simulink model "N3Z_tonetestNotWorking"  (R2014b)
settings: Solver=ode3  SolverMode=SingleTasking  StartTime=0.0  StopTime=1e-4  FixedStep=fpgaclk  RelTol=1e-3
PreLoadFcn:
  | %fpgaclk=1/32.768e6
  | fpgaclk=1/49.162e6
  | 
  | SerialData=[1,zeros(1,11),1,0,0,1]
  | load ../N3workingG/window
  | win=win';  %Go back to using flatter and wider windowed sync function
  | %load ../N3workingG/hanning    %use Hahn window
  | 
  | load ../N3workingG/PREemphasis   %For pre-empasis and deemphasis FIRs
  | 
  | %LUT3=xls2LUT2('../IQI_Qdemod.xls'); LUT3
  | load ../N3workingG/LUT3
  | load ../N3workingG/FIRiq2
  | % xls2LUT
  | 
  | GetProgFiles
  | 
  | PinAssignments    %Get Pin references for TE0722
  | 
  | 
  | 
  | 
  | 
  | %LCD
  | LCDdata=[LCD_D7,LCD_D6,LCD_D5,LCD_D4,LCD_D3,LCD_D2,LCD_D1,LCD_D0] %Note MSB...LSB!
  | LCDctrl=[LCD_E,LCD_RW,LCD_RS];
  | 
  | %for RS232 on pins 3 and 5 of USBB
  | 
  | %BT chip connections for WT12
  | 
  | RX_BT=RXD
  | TX_BT=TXD
  | 
  | RST_BB=RES
  | 
  | %PCMC=PCMC
  | %PCMS=PCMS
  | %PCMI=PCMI
  | %PCMO=PCMO
  | 
  | %Aliases:
  | SRDBT=PCMI
  | STDBT=PCMO
  | SCLK_BT=PCMC
  | SFS_BT=PCMS
  | 
  | %ADC control
  | 
  | %SDOA=SDOA
  | %SDOB=SDOB
  | %SCK=SCK
  | CONV=Csbar
  | CAL=Cal
  | 
  | ADC_G=[ADC_G3,ADC_G2,ADC_G1,ADC_G0]
  | %PD settings hard coded now
  | 
  | %%%%%%
  | TX_LOW=TX_Low
  | ... (+11 lines)
StartFcn:
  | SerialData=[1,zeros(1,11),1,0,0,1]
values from neighbouring files (symbols this model uses):
  ADC_G0 = {'P10'}    [PinAssignments.m]
  ADC_G1 = {'P11'}    [PinAssignments.m]
  ADC_G2 = {'N14'}    [PinAssignments.m]
  ADC_G3 = {'M11'}    [PinAssignments.m]
  Cal = {'L12'}    [PinAssignments.m]
  Csbar = {'M12'}    [PinAssignments.m]
  LCD_D0 = {'J13'}    [PinAssignments.m]
  LCD_D1 = {'J14'}    [PinAssignments.m]
  LCD_D2 = {'F15'}    [PinAssignments.m]
  LCD_D3 = {'H14'}    [PinAssignments.m]
  LCD_D4 = {'G12'}    [PinAssignments.m]
  LCD_D5 = {'L15'}    [PinAssignments.m]
  LCD_D6 = {'M14'}    [PinAssignments.m]
  LCD_D7 = {'K15'}    [PinAssignments.m]
  PCMC = {'H11'}    [PinAssignments.m]
  PCMI = {'H12'}    [PinAssignments.m]
  PCMO = {'N13'}    [PinAssignments.m]
  PCMS = {'M10'}    [PinAssignments.m]
  RES = {'G11'}    [PinAssignments.m]
  RXD = {'H13'}    [PinAssignments.m]
  TX_Low = {'P15'}    [PinAssignments.m]
  TXD = {'P13'}    [PinAssignments.m]
undefined symbols (not defined in the file or in its folder): AXI4, FIRRX, FIRTX, Lite
libraries: xbsIndex_r4 x1238, MyFunctions x43
(part 4 of 9)

== system N3Z_tonetestNotWorking/ADCRead/Subsystem1 ==
  note: April 09, increased delay to latch ADC value to get another bit?
  SDOA : Inport
  Trig : Inport  Port=2
  SDOB : Inport  Port=3
  Concat : xbsIndex_r4/Concat  num_inputs=2  dbl_ovrd=off  block_type=concat
      settings: block_version=VER_STRING_GOES_HERE
  Concat1 : xbsIndex_r4/Concat  num_inputs=2  dbl_ovrd=off  block_type=concat
      settings: block_version=VER_STRING_GOES_HERE
  Convert : xbsIndex_r4/Convert  gui_display_data_type=Fixed-point  arith_type=Boolean  n_bits=8  bin_pt=6  float_type=Single  exp_bits=8  fraction_bits=24  quantization=Truncate  overflow=Wrap  en=off  latency=0  pipeline=off  dbl_ovrd=off  block_type=convert
      settings: xl_area=[0 0 0 0 0 0 0]  block_version=VER_STRING_GOES_HERE
  Delay1 : xbsIndex_r4/Delay  rst=off  infoeditControl=Selection of Reset will increase slice count due to use of real FFs and instead of SRLs  en=off  latency=1  reg_retiming=off  dbl_ovrd=off  block_type=delay
      settings: infoedit=Hardware notes: A delay line is a chain, each link of which is an SRL16 followed by a flip-flop. If register retiming is enabled, the delay line is a chain of flip-flops.  xl_area=[1 1 0 0 0 0 0]  block_version=VER_STRING_GOES_HERE
  Delay3 : xbsIndex_r4/Delay  rst=off  infoeditControl=Selection of Reset will increase slice count due to use of real FFs and instead of SRLs  en=off  latency=1  reg_retiming=off  dbl_ovrd=off  block_type=delay
      settings: infoedit=Hardware notes: A delay line is a chain, each link of which is an SRL16 followed by a flip-flop. If register retiming is enabled, the delay line is a chain of flip-flops.  xl_area=[1 1 0 0 0 0 0]  block_version=VER_STRING_GOES_HERE
  Delay4 : xbsIndex_r4/Delay  rst=off  infoeditControl=Selection of Reset will increase slice count due to use of real FFs and instead of SRLs  en=off  latency=2  reg_retiming=off  dbl_ovrd=off  block_type=delay
      settings: infoedit=Hardware notes: A delay line is a chain, each link of which is an SRL16 followed by a flip-flop. If register retiming is enabled, the delay line is a chain of flip-flops.  xl_area=[1 1 0 0 0 0 0]  block_version=VER_STRING_GOES_HERE
  Delay5 : xbsIndex_r4/Delay  rst=off  infoeditControl=Selection of Reset will increase slice count due to use of real FFs and instead of SRLs  en=off  latency=1  reg_retiming=off  dbl_ovrd=off  block_type=delay
      settings: infoedit=Hardware notes: A delay line is a chain, each link of which is an SRL16 followed by a flip-flop. If register retiming is enabled, the delay line is a chain of flip-flops.  xl_area=[1 1 0 0 0 0 0]  block_version=VER_STRING_GOES_HERE
  Inverter1 : xbsIndex_r4/Inverter  en=off  latency=0  dbl_ovrd=off  block_type=inv
      settings: xl_area=[0 0 0 0 0 0 0]  block_version=VER_STRING_GOES_HERE
  Logical : xbsIndex_r4/Logical  logical_function=AND  inputs=2  en=off  latency=0  precision=Full  arith_type=Unsigned  n_bits=16  bin_pt=0  align_bp=on  dbl_ovrd=off  block_type=logical
      settings: block_version=9.2.01
  Register : xbsIndex_r4/Register  init=0  rst=on  en=on  dbl_ovrd=off  block_type=register
      settings: xl_area=[8 16 0 0 0 0 0]  block_version=VER_STRING_GOES_HERE
  Register1 : xbsIndex_r4/Register  init=0  rst=off  en=on  dbl_ovrd=off  block_type=register
      settings: xl_area=[8 16 0 0 0 0 0]  block_version=VER_STRING_GOES_HERE
  Register2 : xbsIndex_r4/Register  init=0  rst=on  en=on  dbl_ovrd=off  block_type=register
      settings: xl_area=[8 16 0 0 0 0 0]  block_version=VER_STRING_GOES_HERE
  Register3 : xbsIndex_r4/Register  init=0  rst=off  en=on  dbl_ovrd=off  block_type=register
      settings: xl_area=[8 16 0 0 0 0 0]  block_version=VER_STRING_GOES_HERE
  SCKgenerator : Subsystem
  Slice : xbsIndex_r4/Slice  nbits=15  boolean_output=off  mode=Lower Bit Location + Width  bit1=0  base1=MSB of Input  bit0=0  base0=LSB of Input  dbl_ovrd=off  block_type=slice
      settings: block_version=VER_STRING_GOES_HERE
  Slice1 : xbsIndex_r4/Slice  nbits=15  boolean_output=off  mode=Lower Bit Location + Width  bit1=0  base1=MSB of Input  bit0=0  base0=LSB of Input  dbl_ovrd=off  block_type=slice
      settings: infoedit="Extracts a given range of bits from each input sample and presents it at the output.  The output type is ordinarily unsigned with binary point at zero, but can be Boolean when the slice is one bit wide.<P><P>Hardware notes: In hardware this block costs nothing."  block_version=VER_STRING_GOES_HERE
  ADCValueA : Outport
  Conv : Outport  Port=2
  SCK : Outport  Port=3
  DataReady : Outport  Port=4
  ADCValueB : Outport  Port=5
  wires:
  Register/1 -> Slice/1
  Slice/1 -> Concat/1
  Concat/1 -> Register/1, Register1/1
  Convert/1 -> Register/2, Register2/2
  Register1/1 -> ADCValueA/1
  Delay1/1 -> DataReady/1, Register1/2, Register3/2
  Inverter1/1 -> Delay4/1
  Logical/1 -> Register/3, Register2/3
  SCKgenerator/4(DataValid) -> Logical/2
  Delay3/1 -> Convert/1, Conv/1
  Delay4/1 -> Logical/1, SCK/1
  Delay5/1 -> Delay3/1
  SCKgenerator/1(DataReady) -> Delay1/1
  SCKgenerator/2(SCK) -> Inverter1/1
  SCKgenerator/3(Conv) -> Delay5/1
  Trig/1 -> SCKgenerator/1(Trig)
  SDOA/1 -> Concat/2
  Register2/1 -> Slice1/1
  Slice1/1 -> Concat1/1
  Concat1/1 -> Register2/1, Register3/1
  Register3/1 -> ADCValueB/1
  SDOB/1 -> Concat1/2

== system N3Z_tonetestNotWorking/DSProcessor1/Buffer ==
  note: When code is < 128, then code is valid ie buffer not empty.
  Cmd : Inport
  NewCmd : Inport  Port=2
  AckFifo : Inport  Port=3
  Concat : xbsIndex_r4/Concat  num_inputs=2  dbl_ovrd=off  block_type=concat
      settings: block_version=8.2.02
  Convert2 : xbsIndex_r4/Convert  gui_display_data_type=Fixed-point  arith_type=Boolean  n_bits=16  bin_pt=0  float_type=Single  exp_bits=8  fraction_bits=24  quantization=Truncate  overflow=Wrap  en=off  latency=0  pipeline=off  dbl_ovrd=off  block_type=convert
      settings: xl_area=[0, 0, 0, 0, 0, 0, 0]  block_version=VER_STRING_GOES_HERE
  Delay : xbsIndex_r4/Delay  rst=off  infoeditControl=Selection of Reset will increase slice count due to use of real FFs and instead of SRLs  en=off  latency=2  reg_retiming=off  dbl_ovrd=off  block_type=delay
      settings: infoedit=Hardware notes: A delay line is a chain, each link of which is an SRL16 followed by a flip-flop. If register retiming is enabled, the delay line is a chain of flip-flops.  block_version=8.2.02
  FIFO : xbsIndex_r4/FIFO  mem_type=Distributed RAM  performance_options=Standard_FIFO  embedded_registers=off  depth=16  percent_nbits=1  rst=off  rst_latency=1  en=off  use_dcount=off  use_percent_full_port=on  use_almost_empty=off  almost_empty_thresh=2  use_almost_full=off  almost_full_thresh=14  explicit_period=off  dbl_ovrd=off  block_type=fifo
      settings: block_version=8.2.02
  Slice : xbsIndex_r4/Slice  nbits=7  boolean_output=off  mode=Lower Bit Location + Width  bit1=0  base1=MSB of Input  bit0=0  base0=LSB of Input  dbl_ovrd=off  block_type=slice
      settings: infoedit="Extracts a given range of bits from each input sample and presents it at the output.  The output type is ordinarily unsigned with binary point at zero, but can be Boolean when the slice is one bit wide.<P><P>Hardware notes: In hardware this block costs nothing."  block_version=8.2.02
  CmdOut : Outport
  tag scope: User2DSPFIFOfull=global
  wires:
  Cmd/1 -> FIFO/1
  NewCmd/1 -> Delay/1
  Slice/1 -> Concat/2
  FIFO/1 -> Slice/1
  Concat/1 -> CmdOut/1
  FIFO/2 -> Concat/1
  Delay/1 -> FIFO/2
  AckFifo/1 -> Convert2/1
  Convert2/1 -> FIFO/3
  FIFO/4 -> [User2DSPFIFOfull]

== system N3Z_tonetestNotWorking/DSProcessor1/InputSelect ==
  note: 28/2/15 shifted an extra bit down (bottom 16 bits)
      | 17/4/17 use top 16 bits (ie 2 bits higher)
  Select : Inport
  Signal : Inport  Port=2
  strobe : Inport  Port=3
  Cmd : Inport  Port=4
  MultOut : Inport  Port=5
  BTaudioIN : Inport  Port=6
  RAMdata : Inport  Port=7
  Status : Inport  Port=8
  StartToneAmp : Inport  Port=9
  Concat : xbsIndex_r4/Concat  num_inputs=2  dbl_ovrd=off  block_type=concat
      settings: block_version=9.2.01
  Constant : xbsIndex_r4/Constant  const=0  gui_display_data_type=Fixed-point  arith_type=Unsigned  n_bits=7  bin_pt=0  preci_type=Single  exp_width=8  frac_width=24  explicit_period=on  period=fpgaclk  equ=P=C  opselect=C  inp2=PCIN>>17  opr=+  inp1=P  carry=CIN  dbl_ovrd=off  block_type=constant
  Mux : xbsIndex_r4/Mux  inputs=12  en=off  latency=1  precision=Full  arith_type=Unsigned  n_bits=16  bin_pt=14  quantization=Truncate  overflow=Wrap  dbl_ovrd=off  block_type=mux
      settings: block_version=12.2
  Reinterpret1 : xbsIndex_r4/Reinterpret  force_arith_type=on  arith_type=Unsigned  force_bin_pt=on  bin_pt=0  block_type=cast
      settings: block_version=VER_STRING_GOES_HERE
  Slice1 : xbsIndex_r4/Slice  nbits=8  boolean_output=off  mode=Upper Bit Location + Width  bit1=0  base1=MSB of Input  bit0=0  base0=LSB of Input  dbl_ovrd=off  block_type=slice
      settings: block_version=VER_STRING_GOES_HERE
  Slice13 : xbsIndex_r4/Slice  nbits=8  boolean_output=off  mode=Upper Bit Location + Width  bit1=0  base1=MSB of Input  bit0=0  base0=LSB of Input  dbl_ovrd=off  block_type=slice
      settings: block_version=VER_STRING_GOES_HERE
  Slice14 : xbsIndex_r4/Slice  nbits=8  boolean_output=off  mode=Upper Bit Location + Width  bit1=-8  base1=MSB of Input  bit0=0  base0=LSB of Input  dbl_ovrd=off  block_type=slice
      settings: block_version=VER_STRING_GOES_HERE
  Slice2 : xbsIndex_r4/Slice  nbits=8  boolean_output=off  mode=Upper Bit Location + Width  bit1=-8  base1=MSB of Input  bit0=0  base0=LSB of Input  dbl_ovrd=off  block_type=slice
      settings: block_version=VER_STRING_GOES_HERE
  Slice3 : xbsIndex_r4/Slice  nbits=8  boolean_output=off  mode=Upper Bit Location + Width  bit1=-2  base1=MSB of Input  bit0=8  base0=LSB of Input  dbl_ovrd=off  block_type=slice
      settings: block_version=VER_STRING_GOES_HERE
  Slice4 : xbsIndex_r4/Slice  nbits=8  boolean_output=off  mode=Upper Bit Location + Width  bit1=-8-2  base1=MSB of Input  bit0=0  base0=LSB of Input  dbl_ovrd=off  block_type=slice
      settings: block_version=VER_STRING_GOES_HERE
  Slice6 : xbsIndex_r4/Slice  nbits=8  boolean_output=off  mode=Lower Bit Location + Width  bit1=0  base1=MSB of Input  bit0=8  base0=LSB of Input  dbl_ovrd=off  block_type=slice
      settings: block_version=VER_STRING_GOES_HERE
  Slice7 : xbsIndex_r4/Slice  nbits=8  boolean_output=off  mode=Lower Bit Location + Width  bit1=-8  base1=MSB of Input  bit0=0  base0=LSB of Input  dbl_ovrd=off  block_type=slice
      settings: block_version=VER_STRING_GOES_HERE
  Out1 : Outport
  wires:
  Reinterpret1/1 -> Slice3/1, Slice4/1
  Slice3/1 -> Mux/2
  Slice4/1 -> Mux/3
  Signal/1 -> Reinterpret1/1
  Select/1 -> Mux/1
  Mux/1 -> Out1/1
  MultOut/1 -> Slice14/1, Slice13/1
  strobe/1 -> Concat/2
  Concat/1 -> Mux/4
  BTaudioIN/1 -> Slice1/1, Slice2/1
  RAMdata/1 -> Slice6/1, Slice7/1
  Status/1 -> Mux/12
  Cmd/1 -> Mux/5
  Slice13/1 -> Mux/6
  Slice14/1 -> Mux/7
  Slice1/1 -> Mux/8
  Slice2/1 -> Mux/9
  Slice6/1 -> Mux/10
  Slice7/1 -> Mux/11
  Constant/1 -> Concat/1
  StartToneAmp/1 -> Mux/13

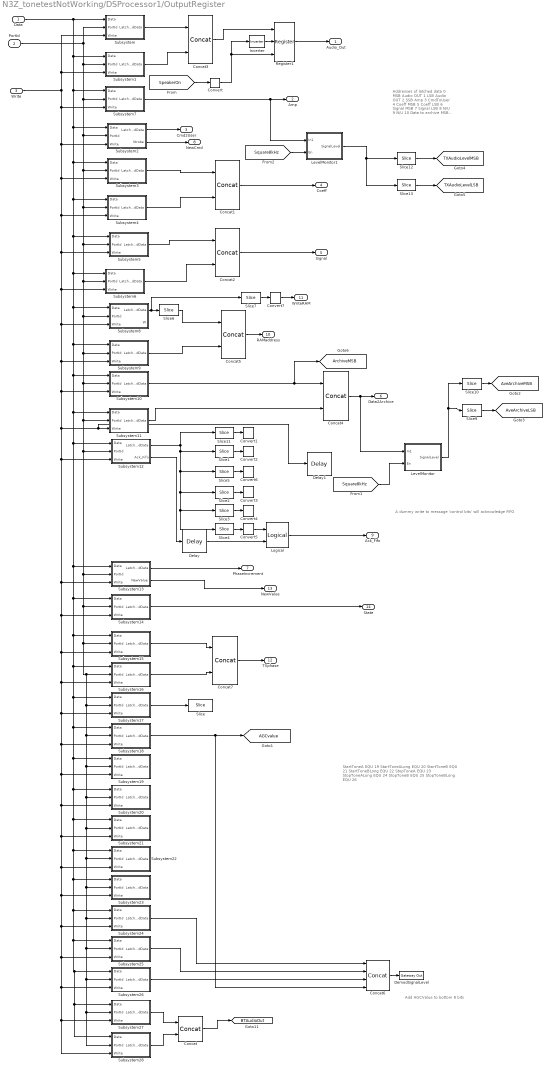
== system N3Z_tonetestNotWorking/DSProcessor1/OutputRegister ==
  note: Add AGCValue to bottom 8 bits
  note: A dummy write to message 'control bits' will acknowledge FIFO
  note: Addresses of latched data
      | 0 MSB Audio OUT
      | 1 LSB Audio OUT
      | 2 SSB Amp
      | 3 CmdToUser
      | 4 Coeff MSB
      | 5 Coeff LSB
      | 6 Signal MSB
      | 7 Signal LSB
      | 8 N/U
      | 9 N/U
      | 10 Data to archive MSB
      | 11 Data to archive LSB
      | 12 Control bits:
      | 	0
      | 	1
      | 	2
      | 	3
      | 	4
      | 	5 Ack Fifo
      |
      | 13 Audio Freq MSB
  note: StartToneA		EQU	19
      | StartToneALong		EQU	20
      | StartToneB		EQU	21
      | StartToneBLong		EQU	22
      | StopToneA		EQU	23
      | StopToneALong		EQU	24
      | StopToneB		EQU	25
      | StopToneBLong		EQU	26
  Data : Inport
  PortId : Inport  Port=2
  Write : Inport  Port=3
  Concat{,1..5,7} (7 alike) : xbsIndex_r4/Concat  num_inputs=2  dbl_ovrd=off  block_type=concat
      Concat1 settings: block_version=8.2.02
      Concat2 settings: block_version=8.2.02
      Concat3 settings: block_version=8.2.02
      Concat4 settings: block_version=8.2.02
      Concat5 settings: block_version=8.2.02
      Concat7 settings: block_version=8.2.02
  Concat6 : xbsIndex_r4/Concat  num_inputs=4  dbl_ovrd=off  block_type=concat
  Convert : xbsIndex_r4/Convert  gui_display_data_type=Boolean  arith_type=Boolean  n_bits=16  bin_pt=14  float_type=Single  exp_bits=8  fraction_bits=24  quantization=Truncate  overflow=Wrap  en=off  latency=0  pipeline=off  dbl_ovrd=off  block_type=convert
  Convert{1..7} (7 alike) : xbsIndex_r4/Convert  gui_display_data_type=Fixed-point  arith_type=Boolean  n_bits=16  bin_pt=0  float_type=Single  exp_bits=8  fraction_bits=24  quantization=Truncate  overflow=Wrap  en=off  latency=0  pipeline=off  dbl_ovrd=off  block_type=convert
      settings: xl_area=[0, 0, 0, 0, 0, 0, 0]  block_version=VER_STRING_GOES_HERE
  Delay : xbsIndex_r4/Delay  rst=off  infoeditControl=Selection of Reset will increase slice count due to use of real FFs and instead of SRLs  en=off  latency=1  reg_retiming=off  dbl_ovrd=off  block_type=delay
      settings: infoedit=Hardware notes: A delay line is a chain, each link of which is an SRL16 followed by a flip-flop. If register retiming is enabled, the delay line is a chain of flip-flops.  block_version=8.2.02
  Delay1 : xbsIndex_r4/Delay  rst=off  infoeditControl=Selection of Reset will increase slice count due to use of real FFs and instead of SRLs  en=off  latency=3  reg_retiming=off  dbl_ovrd=off  block_type=delay
      settings: block_version=8.2.02
  DemodSignalLevel : xbsIndex_r4/Gateway Out  inherit_from_input=off  hdl_port=on  rows=1  columns=1  UseAsDAC=off  DACChannel='1'  interface=AXI4-Lite  automatic_assignment=on  address_offset=hex2dec('00')  intf_name=''  intf_description=''  timing_constraint=None  locs_specified=off  LOCs={}  io_standard={}  block_type=gatewayout
  Inverter : xbsIndex_r4/Inverter  en=off  latency=0  dbl_ovrd=off  block_type=inv
  LevelMonitor : Subsystem
  LevelMonitor1 : Subsystem
  Logical : xbsIndex_r4/Logical  logical_function=AND  inputs=2  en=off  latency=0  precision=Full  arith_type=Unsigned  n_bits=16  bin_pt=0  align_bp=on  dbl_ovrd=off  block_type=logical
      settings: block_version=8.2.02
  Register1 : xbsIndex_r4/Register  init=0  rst=on  en=on  dbl_ovrd=off  block_type=register
      settings: xl_area=[4 8 0 0 0 0 0]  block_version=VER_STRING_GOES_HERE
  Slice : xbsIndex_r4/Slice  nbits=1  boolean_output=off  mode=Lower Bit Location + Width  bit1=0  base1=MSB of Input  bit0=0  base0=LSB of Input  dbl_ovrd=off  block_type=slice
  Slice1 : xbsIndex_r4/Slice  nbits=1  boolean_output=off  mode=Lower Bit Location + Width  bit1=-16  base1=MSB of Input  bit0=1  base0=LSB of Input  dbl_ovrd=off  block_type=slice
      settings: infoedit="Extracts a given range of bits from each input sample and presents it at the output.  The output type is ordinarily unsigned with binary point at zero, but can be Boolean when the slice is one bit wide.<P><P>Hardware notes: In hardware this block costs nothing."  block_version=VER_STRING_GOES_HERE
  Slice10 : xbsIndex_r4/Slice  nbits=8  boolean_output=off  mode=Upper Bit Location + Width  bit1=0  base1=MSB of Input  bit0=0  base0=LSB of Input  dbl_ovrd=off  block_type=slice
      settings: block_version=VER_STRING_GOES_HERE
  Slice11 : xbsIndex_r4/Slice  nbits=1  boolean_output=off  mode=Lower Bit Location + Width  bit1=-16  base1=MSB of Input  bit0=0  base0=LSB of Input  dbl_ovrd=off  block_type=slice
      settings: block_version=VER_STRING_GOES_HERE
  Slice12 : xbsIndex_r4/Slice  nbits=8  boolean_output=off  mode=Upper Bit Location + Width  bit1=0  base1=MSB of Input  bit0=0  base0=LSB of Input  dbl_ovrd=off  block_type=slice
      settings: block_version=VER_STRING_GOES_HERE
  Slice13 : xbsIndex_r4/Slice  nbits=8  boolean_output=off  mode=Lower Bit Location + Width  bit1=-16  base1=MSB of Input  bit0=0  base0=LSB of Input  dbl_ovrd=off  block_type=slice
      settings: block_version=VER_STRING_GOES_HERE
  Slice2 : xbsIndex_r4/Slice  nbits=1  boolean_output=off  mode=Lower Bit Location + Width  bit1=-16  base1=MSB of Input  bit0=3  base0=LSB of Input  dbl_ovrd=off  block_type=slice
      settings: infoedit="Extracts a given range of bits from each input sample and presents it at the output.  The output type is ordinarily unsigned with binary point at zero, but can be Boolean when the slice is one bit wide.<P><P>Hardware notes: In hardware this block costs nothing."  block_version=VER_STRING_GOES_HERE
  Slice3 : xbsIndex_r4/Slice  nbits=1  boolean_output=off  mode=Lower Bit Location + Width  bit1=-16  base1=MSB of Input  bit0=4  base0=LSB of Input  dbl_ovrd=off  block_type=slice
      settings: infoedit="Extracts a given range of bits from each input sample and presents it at the output.  The output type is ordinarily unsigned with binary point at zero, but can be Boolean when the slice is one bit wide.<P><P>Hardware notes: In hardware this block costs nothing."  block_version=VER_STRING_GOES_HERE
  Slice4 : xbsIndex_r4/Slice  nbits=1  boolean_output=off  mode=Lower Bit Location + Width  bit1=-16  base1=MSB of Input  bit0=5  base0=LSB of Input  dbl_ovrd=off  block_type=slice
      settings: block_version=VER_STRING_GOES_HERE
  Slice5 : xbsIndex_r4/Slice  nbits=1  boolean_output=off  mode=Lower Bit Location + Width  bit1=-16  base1=MSB of Input  bit0=2  base0=LSB of Input  dbl_ovrd=off  block_type=slice
      settings: infoedit="Extracts a given range of bits from each input sample and presents it at the output.  The output type is ordinarily unsigned with binary point at zero, but can be Boolean when the slice is one bit wide.<P><P>Hardware notes: In hardware this block costs nothing."  block_version=VER_STRING_GOES_HERE
  Slice6 : xbsIndex_r4/Slice  nbits=2  boolean_output=off  mode=Lower Bit Location + Width  bit1=-16  base1=MSB of Input  bit0=0  base0=LSB of Input  dbl_ovrd=off  block_type=slice
      settings: block_version=VER_STRING_GOES_HERE
  Slice7 : xbsIndex_r4/Slice  nbits=1  boolean_output=off  mode=Lower Bit Location + Width  bit1=-16  base1=MSB of Input  bit0=2  base0=LSB of Input  dbl_ovrd=off  block_type=slice
      settings: block_version=VER_STRING_GOES_HERE
  Slice9 : xbsIndex_r4/Slice  nbits=8  boolean_output=off  mode=Lower Bit Location + Width  bit1=-16  base1=MSB of Input  bit0=0  base0=LSB of Input  dbl_ovrd=off  block_type=slice
      settings: block_version=VER_STRING_GOES_HERE
  Subsystem : Subsystem
  Subsystem1 : Subsystem
  Subsystem10 : Subsystem
  Subsystem11 : Subsystem
  Subsystem12 : Subsystem
  Subsystem13 : Subsystem
  Subsystem14 : Subsystem
  Subsystem15 : Subsystem
  Subsystem16 : Subsystem
  Subsystem17 : Subsystem
  Subsystem18 : Subsystem
  Subsystem19 : Subsystem
  Subsystem2 : Subsystem
  Subsystem20 : Subsystem
  Subsystem21 : Subsystem
  Subsystem22 : Subsystem
  Subsystem23 : Subsystem
  Subsystem24 : Subsystem
  Subsystem25 : Subsystem
  Subsystem26 : Subsystem
  Subsystem27 : Subsystem
  Subsystem28 : Subsystem
  Subsystem3 : Subsystem
  Subsystem4 : Subsystem
  Subsystem5 : Subsystem
  Subsystem6 : Subsystem
  Subsystem7 : Subsystem
  Subsystem8 : Subsystem
  Subsystem9 : Subsystem
  Audio_Out : Outport
  Amp : Outport  Port=2
  Cmd2User : Outport  Port=3
  Coeff : Outport  Port=4
  Signal : Outport  Port=5
  Data2Archive : Outport  Port=6
  PhaseIncrement : Outport  Port=7
  NewCmd : Outport  Port=8
  Ack_Fifo : Outport  Port=9
  RAMaddress : Outport  Port=10
  WriteRAM : Outport  Port=11
  TXphase : Outport  Port=12
  NewValue : Outport  Port=13
  State : Outport  Port=14
  tag scope: AGCvalue=global, ArchiveMSB=global, AveArchiveLSB=global, AveArchiveMSB=global, BTAudioOut=global, TXAudioLevelLSB=global, TXAudioLevelMSB=global
  wires:
  PortId/1 -> Subsystem/2(PortId), Subsystem1/2(PortId), Subsystem7/2(PortId), Subsystem2/2(PortId), Subsystem3/2(PortId), Subsystem4/2(PortId), Subsystem5/2(PortId), Subsystem6/2(PortId), Subsystem8/2(PortId), Subsystem9/2(PortId), Subsystem10/2(PortId), Subsystem11/2(PortId), Subsystem12/2(PortId), Subsystem13/2(PortId), Subsystem14/2(PortId), Subsystem15/2(PortId), Subsystem16/2(PortId), Subsystem17/2(PortId), Subsystem18/2(PortId), Subsystem19/2(PortId), Subsystem20/2(PortId), Subsystem21/2(PortId), Subsystem22/2(PortId), Subsystem23/2(PortId), Subsystem24/2(PortId), Subsystem25/2(PortId), Subsystem28/2(PortId), Subsystem27/2(PortId), Subsystem26/2(PortId)
  Data/1 -> Subsystem/1(Data), Subsystem1/1(Data), Subsystem7/1(Data), Subsystem2/1(Data), Subsystem3/1(Data), Subsystem4/1(Data), Subsystem5/1(Data), Subsystem6/1(Data), Subsystem8/1(Data), Subsystem9/1(Data), Subsystem10/1(Data), Subsystem11/1(Data), Subsystem12/1(Data), Subsystem13/1(Data), Subsystem14/1(Data), Subsystem15/1(Data), Subsystem16/1(Data), Subsystem17/1(Data), Subsystem18/1(Data), Subsystem19/1(Data), Subsystem20/1(Data), Subsystem21/1(Data), Subsystem22/1(Data), Subsystem23/1(Data), Subsystem24/1(Data), Subsystem25/1(Data), Subsystem28/1(Data), Subsystem27/1(Data), Subsystem26/1(Data)
  Write/1 -> Subsystem1/3(Write), Subsystem/3(Write), Subsystem2/3(Write), Subsystem3/3(Write), Subsystem4/3(Write), Subsystem5/3(Write), Subsystem6/3(Write), Subsystem8/3(Write), Subsystem9/3(Write), Subsystem10/3(Write), Subsystem12/3(Write), Subsystem13/3(Write), Subsystem14/3(Write), Subsystem15/3(Write), Subsystem16/3(Write), Subsystem17/3(Write), Subsystem18/3(Write), Subsystem19/3(Write), Subsystem20/3(Write), Subsystem21/3(Write), Subsystem22/3(Write), Subsystem23/3(Write), Subsystem24/3(Write), Subsystem25/3(Write), Subsystem27/3(Write), Subsystem28/3(Write), Subsystem26/3(Write), Subsystem11/3(Write), Delay1/1, Subsystem7/3(Write)
  Subsystem2/1(LatchedData) -> Cmd2User/1
  Subsystem/1(LatchedData) -> Concat3/1
  Subsystem1/1(LatchedData) -> Concat3/2
  Subsystem7/1(LatchedData) -> Amp/1, LevelMonitor1/1(In1)
  Concat1/1 -> Coeff/1
  Concat2/1 -> Signal/1
  Subsystem11/1(LatchedData) -> Concat4/2
  Concat4/1 -> Data2Archive/1, LevelMonitor/1(In1)
  Subsystem10/1(LatchedData) -> [ArchiveMSB], Concat4/1
  Subsystem3/1(LatchedData) -> Concat1/1
  Subsystem4/1(LatchedData) -> Concat1/2
  Subsystem5/1(LatchedData) -> Concat2/1
  Subsystem6/1(LatchedData) -> Concat2/2
  Subsystem12/1(LatchedData) -> Slice2/1, Slice3/1, Slice4/1, Slice5/1, Slice1/1, Slice11/1
  Slice4/1 -> Convert5/1
  Convert5/1 -> Logical/1
  Subsystem2/2(Strobe) -> NewCmd/1
  Subsystem12/2(Ack_Fifo) -> Delay/1
  Logical/1 -> Ack_Fifo/1
  Delay/1 -> Logical/2
  Subsystem8/1(LatchedData) -> Slice6/1, Slice7/1
  Subsystem9/1(LatchedData) -> Concat5/2
  Slice11/1 -> Convert1/1
  Slice1/1 -> Convert2/1
  Slice2/1 -> Convert3/1
  Slice3/1 -> Convert4/1
  Slice5/1 -> Convert6/1
  Concat5/1 -> RAMaddress/1
  Slice6/1 -> Concat5/1
  Slice7/1 -> Convert7/1
  Convert7/1 -> WriteRAM/1
  Subsystem13/1(LatchedData) -> PhaseIncrement/1
  Subsystem15/1(LatchedData) -> Concat7/1
  Subsystem16/1(LatchedData) -> Concat7/2
  Concat7/1 -> TXphase/1
  Subsystem13/2(NewValue) -> NewValue/1
  Concat3/1 -> Register1/1
  Register1/1 -> Audio_Out/1
  Subsystem17/1(LatchedData) -> Slice/1
  Subsystem18/1(LatchedData) -> Concat6/4, [AGCvalue]
  Inverter/1 -> Register1/2
  [SpeakerOn] -> Convert/1
  Subsystem24/1(LatchedData) -> Concat6/1
  Subsystem25/1(LatchedData) -> Concat6/2
  Subsystem26/1(LatchedData) -> Concat6/3
  LevelMonitor/1(SignalLevel) -> Slice10/1, Slice9/1
  Slice10/1 -> [AveArchiveMSB]
  Slice9/1 -> [AveArchiveLSB]
  LevelMonitor1/1(SignalLevel) -> Slice12/1, Slice13/1
  Slice12/1 -> [TXAudioLevelMSB]
  Slice13/1 -> [TXAudioLevelLSB]
  [Square8kHz] -> LevelMonitor/2(En)
  [Square8kHz] -> LevelMonitor1/2(En)
  Subsystem14/1(LatchedData) -> State/1
  Subsystem27/1(LatchedData) -> Concat/1
  Subsystem28/1(LatchedData) -> Concat/2
  Concat/1 -> [BTAudioOut]
  Convert/1 -> Inverter/1, Register1/3
  Concat6/1 -> DemodSignalLevel/1

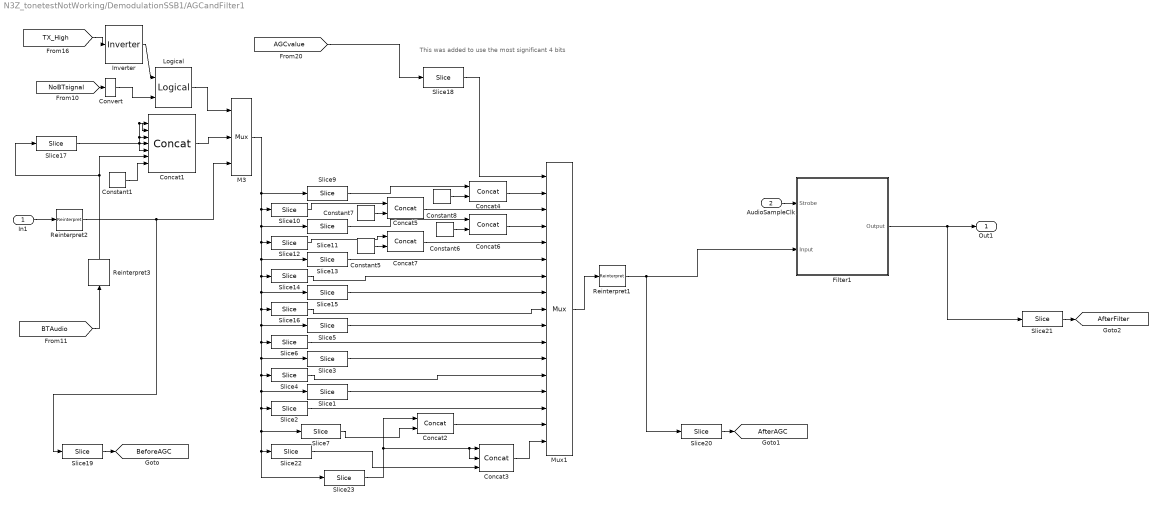
== system N3Z_tonetestNotWorking/DemodulationSSB1/AGCandFilter1 ==
  note: This was added to use the most significant 4 bits
  In1 : Inport
  AudioSampleClk : Inport  Port=2
  Concat1 : xbsIndex_r4/Concat  num_inputs=7  dbl_ovrd=off  block_type=concat
  Concat{2,4..7} (5 alike) : xbsIndex_r4/Concat  num_inputs=2  dbl_ovrd=off  block_type=concat
  Concat3 : xbsIndex_r4/Concat  num_inputs=3  dbl_ovrd=off  block_type=concat
  Constant1 : xbsIndex_r4/Constant  const=0  gui_display_data_type=Fixed-point  arith_type=Unsigned  n_bits=4  bin_pt=0  preci_type=Single  exp_width=8  frac_width=24  explicit_period=on  period=fpgaclk  equ=P=C  opselect=C  inp2=PCIN>>17  opr=+  inp1=P  carry=CIN  dbl_ovrd=off  block_type=constant
  Constant5 : xbsIndex_r4/Constant  const=0  gui_display_data_type=Fixed-point  arith_type=Unsigned  n_bits=1  bin_pt=0  preci_type=Single  exp_width=8  frac_width=24  explicit_period=on  period=fpgaclk  equ=P=C  opselect=C  inp2=PCIN>>17  opr=+  inp1=P  carry=CIN  dbl_ovrd=off  block_type=constant
  Constant6 : xbsIndex_r4/Constant  const=0  gui_display_data_type=Fixed-point  arith_type=Unsigned  n_bits=2  bin_pt=0  preci_type=Single  exp_width=8  frac_width=24  explicit_period=on  period=fpgaclk  equ=P=C  opselect=C  inp2=PCIN>>17  opr=+  inp1=P  carry=CIN  dbl_ovrd=off  block_type=constant
  Constant7 : xbsIndex_r4/Constant  const=0  gui_display_data_type=Fixed-point  arith_type=Unsigned  n_bits=3  bin_pt=0  preci_type=Single  exp_width=8  frac_width=24  explicit_period=on  period=fpgaclk  equ=P=C  opselect=C  inp2=PCIN>>17  opr=+  inp1=P  carry=CIN  dbl_ovrd=off  block_type=constant
  Constant8 : xbsIndex_r4/Constant  const=0  gui_display_data_type=Fixed-point  arith_type=Unsigned  n_bits=4  bin_pt=0  preci_type=Single  exp_width=8  frac_width=24  explicit_period=on  period=fpgaclk  equ=P=C  opselect=C  inp2=PCIN>>17  opr=+  inp1=P  carry=CIN  dbl_ovrd=off  block_type=constant
  Convert : xbsIndex_r4/Convert  gui_display_data_type=Fixed-point  arith_type=Unsigned  n_bits=1  bin_pt=0  float_type=Single  exp_bits=8  fraction_bits=24  quantization=Truncate  overflow=Wrap  en=off  latency=0  pipeline=off  dbl_ovrd=off  block_type=convert
      settings: block_version=8.2.02
  Filter1 : Subsystem
  Inverter : xbsIndex_r4/Inverter  en=off  latency=0  dbl_ovrd=off  block_type=inv
  Logical : xbsIndex_r4/Logical  logical_function=OR  inputs=2  en=off  latency=1  precision=Full  arith_type=Unsigned  n_bits=16  bin_pt=0  align_bp=on  dbl_ovrd=off  block_type=logical
  M3 : xbsIndex_r4/Mux  inputs=2  en=off  latency=1  precision=Full  arith_type=Unsigned  n_bits=16  bin_pt=14  quantization=Truncate  overflow=Wrap  dbl_ovrd=off  block_type=mux
      settings: xl_area=[18 18 0 36 0 0 0]  block_version=8.2.02
  Mux1 : xbsIndex_r4/Mux  inputs=16  en=off  latency=1  precision=Full  arith_type=Unsigned  n_bits=16  bin_pt=14  quantization=Truncate  overflow=Wrap  dbl_ovrd=off  block_type=mux
  Reinterpret1 : xbsIndex_r4/Reinterpret  force_arith_type=on  arith_type="Signed  (2's comp)"  force_bin_pt=on  bin_pt=0  block_type=cast
      settings: block_version=VER_STRING_GOES_HERE
  Reinterpret2 : xbsIndex_r4/Reinterpret  force_arith_type=on  arith_type=Unsigned  force_bin_pt=on  bin_pt=0  block_type=cast
      settings: block_version=VER_STRING_GOES_HERE
  Reinterpret3 : xbsIndex_r4/Reinterpret  force_arith_type=on  arith_type=Unsigned  force_bin_pt=on  bin_pt=0  block_type=cast
      settings: block_version=VER_STRING_GOES_HERE
  Slice1 : xbsIndex_r4/Slice  nbits=16  boolean_output=off  mode=Upper Bit Location + Width  bit1=-1  base1=MSB of Input  bit0=0  base0=LSB of Input  dbl_ovrd=off  block_type=slice
  Slice10 : xbsIndex_r4/Slice  nbits=13  boolean_output=off  mode=Upper Bit Location + Width  bit1=-12  base1=MSB of Input  bit0=0  base0=LSB of Input  dbl_ovrd=off  block_type=slice
  Slice11 : xbsIndex_r4/Slice  nbits=14  boolean_output=off  mode=Upper Bit Location + Width  bit1=-11  base1=MSB of Input  bit0=0  base0=LSB of Input  dbl_ovrd=off  block_type=slice
  Slice12 : xbsIndex_r4/Slice  nbits=15  boolean_output=off  mode=Upper Bit Location + Width  bit1=-10  base1=MSB of Input  bit0=0  base0=LSB of Input  dbl_ovrd=off  block_type=slice
  Slice13 : xbsIndex_r4/Slice  nbits=16  boolean_output=off  mode=Upper Bit Location + Width  bit1=-9  base1=MSB of Input  bit0=0  base0=LSB of Input  dbl_ovrd=off  block_type=slice
  Slice14 : xbsIndex_r4/Slice  nbits=16  boolean_output=off  mode=Upper Bit Location + Width  bit1=-8  base1=MSB of Input  bit0=0  base0=LSB of Input  dbl_ovrd=off  block_type=slice
  Slice15 : xbsIndex_r4/Slice  nbits=16  boolean_output=off  mode=Upper Bit Location + Width  bit1=-7  base1=MSB of Input  bit0=0  base0=LSB of Input  dbl_ovrd=off  block_type=slice
  Slice16 : xbsIndex_r4/Slice  nbits=16  boolean_output=off  mode=Upper Bit Location + Width  bit1=-6  base1=MSB of Input  bit0=0  base0=LSB of Input  dbl_ovrd=off  block_type=slice
  Slice17 : xbsIndex_r4/Slice  nbits=1  boolean_output=off  mode=Upper Bit Location + Width  bit1=0  base1=MSB of Input  bit0=0  base0=LSB of Input  dbl_ovrd=off  block_type=slice
  Slice18 : xbsIndex_r4/Slice  nbits=4  boolean_output=off  mode=Lower Bit Location + Width  bit1=0  base1=MSB of Input  bit0=2  base0=LSB of Input  dbl_ovrd=off  block_type=slice
  Slice19 : xbsIndex_r4/Slice  nbits=8  boolean_output=off  mode=Upper Bit Location + Width  bit1=0  base1=MSB of Input  bit0=0  base0=LSB of Input  dbl_ovrd=off  block_type=slice
  Slice2 : xbsIndex_r4/Slice  nbits=16  boolean_output=off  mode=Upper Bit Location + Width  bit1=0  base1=MSB of Input  bit0=0  base0=LSB of Input  dbl_ovrd=off  block_type=slice
  Slice20 : xbsIndex_r4/Slice  nbits=8  boolean_output=off  mode=Upper Bit Location + Width  bit1=0  base1=MSB of Input  bit0=0  base0=LSB of Input  dbl_ovrd=off  block_type=slice
  Slice21 : xbsIndex_r4/Slice  nbits=8  boolean_output=off  mode=Upper Bit Location + Width  bit1=-2  base1=MSB of Input  bit0=0  base0=LSB of Input  dbl_ovrd=off  block_type=slice
  Slice22 : xbsIndex_r4/Slice  nbits=14  boolean_output=off  mode=Upper Bit Location + Width  bit1=0  base1=MSB of Input  bit0=0  base0=LSB of Input  dbl_ovrd=off  block_type=slice
  Slice23 : xbsIndex_r4/Slice  nbits=1  boolean_output=off  mode=Upper Bit Location + Width  bit1=0  base1=MSB of Input  bit0=0  base0=LSB of Input  dbl_ovrd=off  block_type=slice
  Slice3 : xbsIndex_r4/Slice  nbits=16  boolean_output=off  mode=Upper Bit Location + Width  bit1=-3  base1=MSB of Input  bit0=0  base0=LSB of Input  dbl_ovrd=off  block_type=slice
  Slice4 : xbsIndex_r4/Slice  nbits=16  boolean_output=off  mode=Upper Bit Location + Width  bit1=-2  base1=MSB of Input  bit0=0  base0=LSB of Input  dbl_ovrd=off  block_type=slice
  Slice5 : xbsIndex_r4/Slice  nbits=16  boolean_output=off  mode=Upper Bit Location + Width  bit1=-5  base1=MSB of Input  bit0=0  base0=LSB of Input  dbl_ovrd=off  block_type=slice
  Slice6 : xbsIndex_r4/Slice  nbits=16  boolean_output=off  mode=Upper Bit Location + Width  bit1=-4  base1=MSB of Input  bit0=0  base0=LSB of Input  dbl_ovrd=off  block_type=slice
  Slice7 : xbsIndex_r4/Slice  nbits=15  boolean_output=off  mode=Upper Bit Location + Width  bit1=0  base1=MSB of Input  bit0=0  base0=LSB of Input  dbl_ovrd=off  block_type=slice
  Slice9 : xbsIndex_r4/Slice  nbits=12  boolean_output=off  mode=Upper Bit Location + Width  bit1=-13  base1=MSB of Input  bit0=0  base0=LSB of Input  dbl_ovrd=off  block_type=slice
  Out1 : Outport
  tag scope: AfterAGC=global, AfterFilter=global, BeforeAGC=global
  wires:
  Filter1/1(Output) -> Slice21/1, Out1/1
  Constant6/1 -> Concat6/2
  Constant7/1 -> Concat5/2
  Constant8/1 -> Concat4/2
  Slice23/1 -> Concat2/1, Concat3/2, Concat3/1
  Constant5/1 -> Concat7/2
  Concat7/1 -> Mux1/5
  Concat6/1 -> Mux1/4
  Concat5/1 -> Mux1/3
  Concat4/1 -> Mux1/2
  Slice12/1 -> Concat7/1
  Slice11/1 -> Concat6/1
  Slice10/1 -> Concat5/1
  Slice9/1 -> Concat4/1
  Mux1/1 -> Reinterpret1/1
  AudioSampleClk/1 -> Filter1/1(Strobe)
  Slice3/1 -> Mux1/12
  In1/1 -> Reinterpret2/1
  Slice16/1 -> Mux1/9
  Slice15/1 -> Mux1/8
  Slice14/1 -> Mux1/7
  Slice13/1 -> Mux1/6
  [AGCvalue] -> Slice18/1
  Slice6/1 -> Mux1/11
  Slice5/1 -> Mux1/10
  Slice4/1 -> Mux1/13
  Slice2/1 -> Mux1/15
  Slice1/1 -> Mux1/14
  Reinterpret1/1 -> Slice20/1, Filter1/2(Input)
  [NoBTsignal] -> Convert/1
  [TX_High] -> Inverter/1
  Inverter/1 -> Logical/1
  Logical/1 -> M3/1
  Convert/1 -> Logical/2
  M3/1 -> Slice23/1, Slice22/1, Slice7/1, Slice2/1, Slice1/1, Slice4/1, Slice3/1, Slice6/1, Slice5/1, Slice16/1, Slice15/1, Slice14/1, Slice13/1, Slice12/1, Slice11/1, Slice10/1, Slice9/1
  Reinterpret2/1 -> Slice19/1, M3/3
  Slice17/1 -> Concat1/5, Concat1/4, Concat1/3, Concat1/2, Concat1/1
  [BTAudio] -> Reinterpret3/1
  Constant1/1 -> Concat1/7
  Concat1/1 -> M3/2
  Reinterpret3/1 -> Concat1/6, Slice17/1
  Slice18/1 -> Mux1/1
  Slice19/1 -> [BeforeAGC]
  Slice20/1 -> [AfterAGC]
  Slice21/1 -> [AfterFilter]
  Slice7/1 -> Concat2/2
  Slice22/1 -> Concat3/3
  Concat3/1 -> Mux1/17
  Concat2/1 -> Mux1/16

== system N3Z_tonetestNotWorking/DemodulationSSB1/CtrlBitSequenceAddress ==
  note: Should cycle through steps just once
  Trig : Inport
  Constant : xbsIndex_r4/Constant  const=1  gui_display_data_type=Boolean  arith_type=Boolean  n_bits=16  bin_pt=14  preci_type=Single  exp_width=8  frac_width=24  explicit_period=on  period=fpgaclk  equ=P=C  opselect=C  inp2=PCIN>>17  opr=+  inp1=P  carry=CIN  dbl_ovrd=off  block_type=constant
      settings: block_version=8.2.02
  Constant3 : xbsIndex_r4/Constant  const=31  gui_display_data_type=Fixed-point  arith_type=Unsigned  n_bits=5  bin_pt=0  preci_type=Single  exp_width=8  frac_width=24  explicit_period=on  period=fpgaclk  equ=P=C  opselect=C  inp2=PCIN>>17  opr=+  inp1=P  carry=CIN  dbl_ovrd=off  block_type=constant
      settings: block_version=8.2.02
  Counter2 : xbsIndex_r4/Counter  cnt_type=Free Running  cnt_to=Inf  operation=Up  start_count=0  cnt_by_val=1  arith_type=Unsigned  n_bits=5  bin_pt=0  load_pin=off  rst=on  en=off  explicit_period=on  period=fpgaclk  use_behavioral_HDL=off  implementation=Fabric  use_rpm=off  dbl_ovrd=off  block_type=counter
      settings: xl_area=[4 5 0 5 0 0 0]  block_version=8.2.02
  Register3 : xbsIndex_r4/Register  init=0  rst=on  en=on  dbl_ovrd=off  block_type=register
      settings: xl_area=[1 1 0 0 0 0 0]  block_version=8.2.02
  Relational : xbsIndex_r4/Relational  mode=a=b  op_type=Bool  en=off  latency=1  dbl_ovrd=off  block_type=relational
      settings: xl_area=[2 1 0 3 0 0 0]  block_version=8.2.02
  CtrlSequencerAddress : Outport
  wires:
  Counter2/1 -> Relational/1, CtrlSequencerAddress/1
  Constant3/1 -> Relational/2
  Constant/1 -> Register3/1
  Register3/1 -> Counter2/1
  Relational/1 -> Register3/3
  Trig/1 -> Register3/2

== system N3Z_tonetestNotWorking/DemodulationSSB1/CtrlSequencer ==
  note: Extra bit added to select add or subtract I+/-Q
  In1 : Inport
  BitBasher : xbsIndex_r4/BitBasher  bitexpr=|  display_expr=off  sr_1=1  arith_type1=Unsigned  bin_pt1=0  sr_2=2  arith_type2=Unsigned  bin_pt2=0  sr_3=3  arith_type3=Unsigned  bin_pt3=0  sr_4=4  arith_type4=Unsigned  bin_pt4=0  dbl_ovrd=off  block_type=bitbasher
      | <html><head><meta name="qrichtext" content="1" /></head><body style="font-size:8pt;font-family:MS Shell Dlg">
      | <p>M1={a[0]}<br />M2={a[2:1]}<br />IQaddress={a[3]}<br /></p>
      | </body></html>
      settings: block_version=8.2.02
      settings: infoedit=|
      | Allows
      |      extraction, concatenation and augmentation of bits
  BitBasher1 : xbsIndex_r4/BitBasher  bitexpr=|  display_expr=off  sr_1=1  arith_type1=Unsigned  bin_pt1=0  sr_2=2  arith_type2=Unsigned  bin_pt2=0  sr_3=3  arith_type3=Unsigned  bin_pt3=0  sr_4=4  arith_type4=Unsigned  bin_pt4=0  dbl_ovrd=off  block_type=bitbasher
      | <html><head><meta name="qrichtext" content="1" /></head><body style="font-size:8pt;font-family:MS Shell Dlg">
      | <p>LatchI={a[4]}<br />LatchQ={a[5]}<br />LatchDemod={a[6]}<br /></p>
      | </body></html>
      settings: block_version=8.2.02
      settings: infoedit=|
      | Allows
      |      extraction, concatenation and augmentation of bits
  BitBasher2 : xbsIndex_r4/BitBasher  bitexpr=|  display_expr=off  sr_1=1  arith_type1=Unsigned  bin_pt1=0  sr_2=2  arith_type2=Unsigned  bin_pt2=0  sr_3=3  arith_type3=Unsigned  bin_pt3=0  sr_4=4  arith_type4=Unsigned  bin_pt4=0  dbl_ovrd=off  block_type=bitbasher
      | <!DOCTYPE HTML PUBLIC "-//W3C//DTD HTML 4.0//EN" "http://www.w3.org/TR/REC-html40/strict.dtd">
      | <html><head><meta name="qrichtext" content="1" /><style type="text/css">
      | p, li { white-space: pre-wrap; }
      | </style></head><body style=" font-family:'MS Shell Dlg 2'; font-size:8.25pt; font-weight:400; font-style:normal;">
      | <p style=" margin-top:12px; margin-bottom:12px; margin-left:0px; margin-right:0px; -qt-block-indent:0; text-indent:0px; font-family:'MS Shell Dlg'; font-size:8pt;">Accu={a[7]}<br />Increment={a[8]}<br />IQadd_sub={a[9]}<br /></p></body></html>
      settings: block_version=8.2.02
  Convert{,1..5} (6 alike) : xbsIndex_r4/Convert  gui_display_data_type=Fixed-point  arith_type=Boolean  n_bits=16  bin_pt=14  float_type=Single  exp_bits=8  fraction_bits=24  quantization=Truncate  overflow=Wrap  en=off  latency=0  pipeline=off  dbl_ovrd=off  block_type=convert
      settings: xl_area=[0 0 0 0 0 0 0]  block_version=8.2.02
  CtrlBitSequence : xbsIndex_r4/ROM  depth=32  initVector=LUT3  distributed_mem=Distributed memory  rst=off  init_reg=0  en=off  latency=1  gui_display_data_type=Fixed-point  arith_type=Unsigned  n_bits=10  bin_pt=0  preci_type=Single  exp_width=8  frac_width=24  optimize=Area  use_rpm=on  dbl_ovrd=off  block_type=sprom
      settings: xl_area=[8 9 0 15 0 0 0]  block_version=8.2.02
  M1 : Outport
  M2 : Outport  Port=2
  IQaddress : Outport  Port=3
  LatchI : Outport  Port=4
  LatchQ : Outport  Port=5
  LatchDemod : Outport  Port=6
  Accu : Outport  Port=7
  IncrmntStreamAddress : Outport  Port=8
  AllCtrlBits : Outport  Port=9
  IQadd_sub : Outport  Port=10
  wires:
  CtrlBitSequence/1 -> BitBasher1/1, BitBasher2/1, AllCtrlBits/1, BitBasher/1
  BitBasher1/3 -> Convert2/1
  BitBasher1/1 -> Convert4/1
  BitBasher1/2 -> Convert3/1
  BitBasher2/1 -> Convert1/1
  BitBasher2/2 -> Convert/1
  In1/1 -> CtrlBitSequence/1
  BitBasher/1 -> M1/1
  BitBasher/2 -> M2/1
  BitBasher/3 -> IQaddress/1
  Convert4/1 -> LatchI/1
  Convert3/1 -> LatchQ/1
  Convert2/1 -> LatchDemod/1
  Convert1/1 -> Accu/1
  Convert/1 -> IncrmntStreamAddress/1
  Convert5/1 -> IQadd_sub/1
  BitBasher2/3 -> Convert5/1

== system N3Z_tonetestNotWorking/DemodulationSSB1/FilterStreamIntegration ==
  note: Add 2 more bits to try and stop saturating
  note: Changed back to full 31/7/12!!
  Stream2Accu : Inport
  Accu : Inport  Port=2
  Signal : Inport  Port=3
  Rst : Inport  Port=4
  StreamMaturing : Inport  Port=5
  Accumulator1 : xbsIndex_r4/Accumulator  operation=Add  n_bits=25  overflow=Wrap  scale=1  rst=on  hasbypass=on  infoeditControl=reset for floating point data type must be asserted for a minimum of 2 cycles  en=on  latency=0  msb_inp=100  msb=100  lsb=-100  use_behavioral_HDL=on  implementation=Fabric  dbl_ovrd=off  block_type=accum
      settings: xl_area=[13 25 0 25 0 0 0]  block_version=8.2.02
  Accumulator{2..8} (7 alike) : xbsIndex_r4/Accumulator  operation=Add  n_bits=25  overflow=Wrap  scale=1  rst=on  hasbypass=off  infoeditControl=reset for floating point data type must be asserted for a minimum of 2 cycles  en=on  latency=0  msb_inp=100  msb=100  lsb=-100  use_behavioral_HDL=on  implementation=Fabric  dbl_ovrd=off  block_type=accum
      settings: xl_area=[13 25 0 25 0 0 0]  block_version=8.2.02
  AddSub : xbsIndex_r4/AddSub  mode=Addition or Subtraction  use_carryin=off  use_carryout=off  en=off  latency=0  precision=User Defined  arith_type="Signed  (2's comp)"  n_bits=25  bin_pt=17  quantization=Truncate  overflow=Wrap  use_behavioral_HDL=off  hw_selection=Fabric  pipelined=off  use_rpm=on  dbl_ovrd=off  block_type=addsub
      settings: xl_area=[13 0 0 25 0 0 0]  block_version=8.2.02
  AddSub1 : xbsIndex_r4/AddSub  mode=Subtraction  use_carryin=off  use_carryout=off  en=off  latency=0  precision=User Defined  arith_type=Unsigned  n_bits=3  bin_pt=0  quantization=Truncate  overflow=Wrap  use_behavioral_HDL=off  hw_selection=Fabric  pipelined=off  dbl_ovrd=off  block_type=addsub
      settings: block_version=12.2
  Constant : xbsIndex_r4/Constant  const=0  gui_display_data_type=Fixed-point  arith_type=Signed (2's comp)  n_bits=25  bin_pt=17  preci_type=Single  exp_width=8  frac_width=24  explicit_period=on  period=fpgaclk  equ=P=C  opselect=C  inp2=PCIN>>17  opr=+  inp1=P  carry=CIN  dbl_ovrd=off  block_type=constant
      settings: block_version=8.2.02
  Constant1 : xbsIndex_r4/Constant  const=1  gui_display_data_type=Fixed-point  arith_type=Unsigned  n_bits=2  bin_pt=0  preci_type=Single  exp_width=8  frac_width=24  explicit_period=on  period=fpgaclk  equ=P=C  opselect=C  inp2=PCIN>>17  opr=+  inp1=P  carry=CIN  dbl_ovrd=off  block_type=constant
      settings: block_version=12.2
  Convert : xbsIndex_r4/Convert  gui_display_data_type=Fixed-point  arith_type=Boolean  n_bits=16  bin_pt=14  float_type=Single  exp_bits=8  fraction_bits=24  quantization=Truncate  overflow=Wrap  en=off  latency=0  pipeline=off  dbl_ovrd=off  block_type=convert
      settings: xl_area=[0 0 0 0 0 0 0]  block_version=8.2.02
  Delay : xbsIndex_r4/Delay  rst=off  infoeditControl=Selection of Reset will increase slice count due to use of real FFs and instead of SRLs  en=off  latency=2  reg_retiming=off  dbl_ovrd=off  block_type=delay
      settings: xl_area=[2 3 0 3 0 0 0]  block_version=8.2.02
  Delay1 : xbsIndex_r4/Delay  rst=off  infoeditControl=Selection of Reset will increase slice count due to use of real FFs and instead of SRLs  en=off  latency=1  reg_retiming=off  dbl_ovrd=off  block_type=delay
      settings: infoedit=Hardware notes: A delay line is a chain, each link of which is an SRL16 followed by a flip-flop. If register retiming is enabled, the delay line is a chain of flip-flops.  xl_area=[1 1 0 0 0 0 0]  block_version=8.2.02
  Delay2 : xbsIndex_r4/Delay  rst=off  infoeditControl=Selection of Reset will increase slice count due to use of real FFs and instead of SRLs  en=off  latency=2  reg_retiming=off  dbl_ovrd=off  block_type=delay
      settings: infoedit=Hardware notes: A delay line is a chain, each link of which is an SRL16 followed by a flip-flop. If register retiming is enabled, the delay line is a chain of flip-flops.  xl_area=[2 3 0 3 0 0 0]  block_version=8.2.02
  Delay3 : xbsIndex_r4/Delay  rst=off  infoeditControl=Selection of Reset will increase slice count due to use of real FFs and instead of SRLs  en=off  latency=1  reg_retiming=off  dbl_ovrd=off  block_type=delay
      settings: infoedit=Hardware notes: A delay line is a chain, each link of which is an SRL16 followed by a flip-flop. If register retiming is enabled, the delay line is a chain of flip-flops.  xl_area=[1 1 0 0 0 0 0]  block_version=8.2.02
  Delay4 : xbsIndex_r4/Delay  rst=off  infoeditControl=Selection of Reset will increase slice count due to use of real FFs and instead of SRLs  en=off  latency=14  reg_retiming=off  dbl_ovrd=off  block_type=delay
      settings: infoedit=Hardware notes: A delay line is a chain, each link of which is an SRL16 followed by a flip-flop. If register retiming is enabled, the delay line is a chain of flip-flops.  xl_area=[13 25 0 25 0 0 0]  block_version=8.2.02
  Logical : xbsIndex_r4/Logical  logical_function=XOR  inputs=2  en=off  latency=0  precision=Full  arith_type=Unsigned  n_bits=16  bin_pt=0  align_bp=on  dbl_ovrd=off  block_type=logical
      settings: xl_area=[1 0 0 1 0 0 0]  block_version=8.2.02
  Mux : xbsIndex_r4/Mux  inputs=8  en=off  latency=1  precision=Full  arith_type=Unsigned  n_bits=16  bin_pt=14  quantization=Truncate  overflow=Wrap  dbl_ovrd=off  block_type=mux
      settings: xl_area=[50 25 0 100 0 0 0]  block_version=8.2.02
  Register : xbsIndex_r4/Register  init=0  rst=off  en=on  dbl_ovrd=off  block_type=register
      settings: xl_area=[13 25 0 0 0 0 0]  block_version=8.2.02
  Register6 : xbsIndex_r4/Register  init=0  rst=off  en=on  dbl_ovrd=off  block_type=register
      settings: xl_area=[1 1 0 0 0 0 0]  block_version=8.2.02
  Slice : xbsIndex_r4/Slice  nbits=1  boolean_output=off  mode=Lower Bit Location + Width  bit1=0  base1=MSB of Input  bit0=2  base0=LSB of Input  dbl_ovrd=off  block_type=slice
      settings: block_version=8.2.02
  Slice1 : xbsIndex_r4/Slice  nbits=1  boolean_output=off  mode=Lower Bit Location + Width  bit1=0  base1=MSB of Input  bit0=1  base0=LSB of Input  dbl_ovrd=off  block_type=slice
      settings: block_version=8.2.02
  Slice2 : xbsIndex_r4/Slice  nbits=3  boolean_output=off  mode=Lower Bit Location + Width  bit1=0  base1=MSB of Input  bit0=0  base0=LSB of Input  dbl_ovrd=off  block_type=slice
      settings: block_version=12.2
  TrigDistrib : Subsystem
  TrigDistrib1 : Subsystem
  DemodSignal : Outport
  DemodStrobe : Outport  Port=2
  wires:
  TrigDistrib/1(Out1) -> Accumulator1/3
  TrigDistrib/2(Out2) -> Accumulator2/3
  Stream2Accu/1 -> Delay/1
  TrigDistrib/3(Out3) -> Accumulator3/3
  TrigDistrib/4(Out4) -> Accumulator4/3, Register6/2
  TrigDistrib/5(Out5) -> Accumulator5/3
  TrigDistrib/6(Out6) -> Accumulator6/3
  TrigDistrib/7(Out7) -> Accumulator7/3
  TrigDistrib/8(Out8) -> Accumulator8/3
  Signal/1 -> Accumulator7/1, Accumulator8/1, Accumulator6/1, Accumulator5/1, Accumulator4/1, Accumulator3/1, Accumulator2/1, Accumulator1/1
  Accu/1 -> Delay1/1
  Rst/1 -> TrigDistrib1/1(Trig), Delay3/1
  StreamMaturing/1 -> TrigDistrib1/2(In2), Delay2/1, Slice2/1
  Mux/1 -> Register/1
  Accumulator1/1 -> Mux/2
  Delay/1 -> TrigDistrib/2(In2)
  Delay1/1 -> TrigDistrib/1(Trig)
  TrigDistrib1/8(Out8) -> Accumulator2/2
  TrigDistrib1/1(Out1) -> Accumulator1/2
  TrigDistrib1/2(Out2) -> Accumulator8/2
  TrigDistrib1/3(Out3) -> Accumulator7/2
  TrigDistrib1/4(Out4) -> Accumulator6/2
  TrigDistrib1/5(Out5) -> Accumulator5/2
  TrigDistrib1/6(Out6) -> Accumulator4/2
  TrigDistrib1/7(Out7) -> Accumulator3/2
  Delay2/1 -> Mux/1
  Accumulator8/1 -> Mux/3
  Accumulator7/1 -> Mux/4
  Accumulator6/1 -> Mux/5
  Accumulator5/1 -> Mux/6
  Accumulator4/1 -> Mux/7
  Accumulator3/1 -> Mux/8
  Accumulator2/1 -> Mux/9
  Delay3/1 -> Register/2, DemodStrobe/1
  Constant/1 -> AddSub/1
  Register6/1 -> Convert/1
  Register/1 -> Delay4/1
  AddSub/1 -> DemodSignal/1
  Slice1/1 -> Logical/1
  Slice/1 -> Logical/2
  Logical/1 -> Register6/1
  Delay4/1 -> AddSub/2
  Convert/1 -> AddSub/3
  AddSub1/1 -> Slice1/1, Slice/1
  Slice2/1 -> AddSub1/1
  Constant1/1 -> AddSub1/2
